simulink model "generico_f"  (R2015a)
settings: Solver=ode23tb  StartTime=0.0  StopTime=0.129  FixedStep=Ts  MaxStep=1e-5  RelTol=1e-4
values from neighbouring files (symbols this model uses):
  Tsc = 1/(fsw)    (= 0.0001)    [leer_ensayo_E3_f.m]    (also in leer_ensayo_E4_f.m; leer_ensayo_E5_f.m)
libraries: simulink x6
Description:
  | Three-Phase Asynchronous Drive with Sensor Control
  | 
  | This example shows how to control and analyze the operation of an
  | Asynchronous Machine (ASM) using sensored rotor field-oriented control.
  | The model shows the main electrical circuit, with three additional subsystems
  | containing the controls, measurements, and scopes.  The Controls subsystem
  | contains two controllers: one for the Grid-Side Converter (AC/DC) and one for
  | the Machine-Side Converter (DC/AC).  The Scopes subsystem contains two time
  | scopes: one for the Grid-Side Converter and one for the ASM. When the model
  | is executed, a Spectrum Analyzer opens and displays frequency data for the
  | A-Phase Supply Current.
  | 
  | 
  | 
  | Copyright 2008-2016 The MathWorks, Inc.
settings Model: Creator=MathWorks  LastModifiedBy=54265
settings SolverCC: PositivePriorityOrder=on  InsertRTBMode=Always
settings DataIOCC: FinalStateName=estado_sim  InitialState=estado_sim_ini  LimitDataPoints=off  SaveFinalState=on  SaveFormat=StructureWithTime  SaveOutput=off  SaveTime=off
settings OptimizationCC: ExpressionDepthLimit=2147483647  EfficientMapNaN2IntZero=off
settings DebuggingCC: UnderspecifiedInitializationDetection=Classic  MergeDetectMultiDrivingBlocksExec=none  SolverPrmCheckMsg=warning  MultiTaskRateTransMsg=warning  StateNameClashWarn=warning
settings HardwareCC: TargetLongLongMode=on  TargetIntDivRoundTo=Zero  TargetEndianess=LittleEndian  TargetHWDeviceType=MATLAB Host  ProdEqTarget=off
settings CodeAppCC: MaxIdLength=128
settings GRTTargetCC: CombineOutputUpdateFcns=off  GRTInterface=on

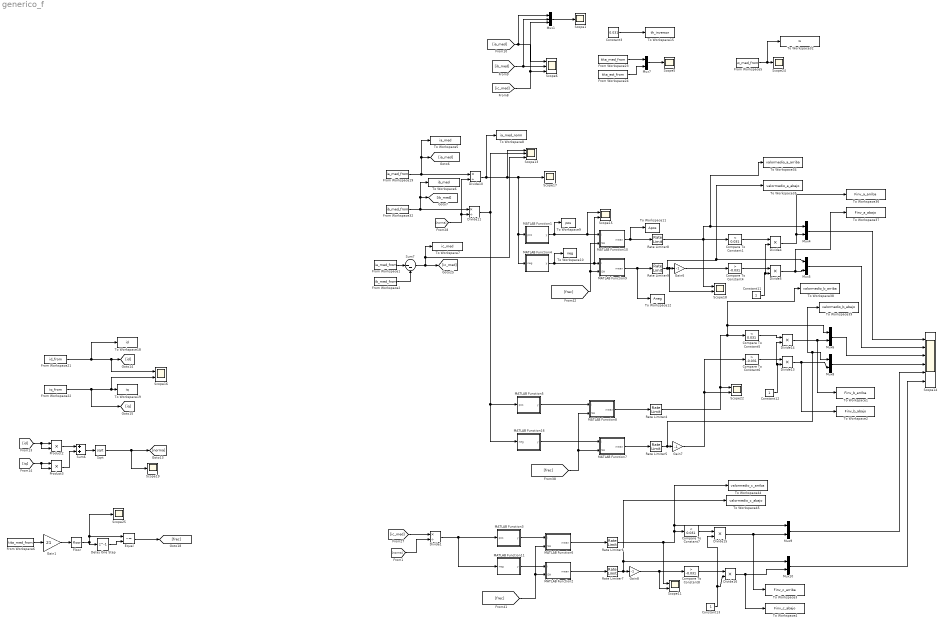
== system generico_f ==
  Compare To Constant1 : simulink/Logic and Bit Operations/Compare To Constant  relop=<  const=0.031  OutDataTypeStr=boolean
  Compare To Constant4 : simulink/Logic and Bit Operations/Compare To Constant  relop=>  const=-0.031  OutDataTypeStr=boolean
  Compare To Constant5 : simulink/Logic and Bit Operations/Compare To Constant  relop=<  const=0.031  OutDataTypeStr=boolean
  Compare To Constant6 : simulink/Logic and Bit Operations/Compare To Constant  relop=>  const=-0.031  OutDataTypeStr=boolean
  Compare To Constant7 : simulink/Logic and Bit Operations/Compare To Constant  relop=<  const=0.031  OutDataTypeStr=boolean
  Compare To Constant8 : simulink/Logic and Bit Operations/Compare To Constant  relop=>  const=-0.031  OutDataTypeStr=boolean
  Constant11 : Constant
  Constant12 : Constant
  Constant13 : Constant
  Constant3 : Constant  Value=0.031
  Delay One Step : Delay  DelayLength=1
  Divide1 : Product  Inputs=*/
  Divide10 : Product  Inputs=*/
  Divide11 : Product  Inputs=*/
  Divide{4..5,13..16} (6 alike) : Product  Inputs=**
  Equal : RelationalOperator  Operator=~=  OutDataTypeStr=boolean
  Floor : Rounding
  From Workspace1 : FromWorkspace  VariableName=ia_med_from  SampleTime=Tsc  OutputAfterFinalValue=Setting to zero
  From Workspace19 : FromWorkspace  VariableName=ia_med_from  SampleTime=Tsc  OutputAfterFinalValue=Setting to zero
  From Workspace2 : FromWorkspace  VariableName=ib_med_from  SampleTime=Tsc  OutputAfterFinalValue=Setting to zero
  From Workspace21 : FromWorkspace  VariableName=id_from  SampleTime=Tsc  OutputAfterFinalValue=Setting to zero
  From Workspace22 : FromWorkspace  VariableName=iq_from  SampleTime=Tsc  OutputAfterFinalValue=Setting to zero
  From Workspace23 : FromWorkspace  VariableName=tita_med_from  SampleTime=Tsc  OutputAfterFinalValue=Setting to zero
  From Workspace24 : FromWorkspace  VariableName=tita_est_from  SampleTime=Tsc  OutputAfterFinalValue=Setting to zero
  From Workspace32 : FromWorkspace  VariableName=ib_med_from  SampleTime=Tsc  OutputAfterFinalValue=Setting to zero
  From Workspace5 : FromWorkspace  VariableName=w_med_from  SampleTime=Tsc  OutputAfterFinalValue=Setting to zero
  From Workspace6 : FromWorkspace  VariableName=tita_med_from  SampleTime=Tsc  OutputAfterFinalValue=Setting to zero
  Gain1 : Gain  Gain=21
  Gain6 : Gain  Gain=-1
  Gain7 : Gain  Gain=-1
  Gain8 : Gain  Gain=-1
  MATLAB Function1 : MATLAB Function  TreatAsAtomicUnit=on
  MATLAB Function10 : MATLAB Function  TreatAsAtomicUnit=on
  MATLAB Function11 : MATLAB Function  TreatAsAtomicUnit=on
  MATLAB Function16 : MATLAB Function  TreatAsAtomicUnit=on
  MATLAB Function2 : MATLAB Function  TreatAsAtomicUnit=on
  MATLAB Function3 : MATLAB Function  TreatAsAtomicUnit=on
  MATLAB Function4 : MATLAB Function  TreatAsAtomicUnit=on
  MATLAB Function5 : MATLAB Function  TreatAsAtomicUnit=on
  MATLAB Function6 : MATLAB Function  TreatAsAtomicUnit=on
  MATLAB Function7 : MATLAB Function  TreatAsAtomicUnit=on
  MATLAB Function8 : MATLAB Function  TreatAsAtomicUnit=on
  MATLAB Function9 : MATLAB Function  TreatAsAtomicUnit=on
  Mux1 : Mux  Inputs=3
  Mux{4..10} (7 alike) : Mux  Inputs=2
  Product2 : Product
  Product3 : Product
  Rate Limiter{4..9} (6 alike) : RateLimiter  RisingSlewLimit=100000  FallingSlewLimit=-40
  Scope{1,5,17,19,24..25} (6 alike) : Scope
      Scope1 settings: TimeRange=1.2  YMin=0.6965  YMax=0.70025
      Scope17 settings: TimeRange=1.2  YMin=-1066.28  YMax=178.833  SaveName=ScopeData22
      Scope19 settings: TimeRange=1.2  YMin=-1066.28418  YMax=178.83301  SaveName=ScopeData21  Decimation=10
      Scope24 settings: TimeRange=0.129  YMin=0.45  YMax=0.55  SaveName=ScopeData28
      Scope25 settings: TimeRange=1.2  YMin=70.17554  YMax=98.54179  SaveName=ScopeData29  Decimation=10
      Scope5 settings: TimeRange=1.2  YMin=0.6965  YMax=0.70025  SaveName=ScopeData4  Decimation=10
  Scope{11,15..16,18,22} (5 alike) : Scope  NumInputPorts=2
      Scope11 settings: TimeRange=1.2  YMin=-1066.28~-5  YMax=178.833~5  SaveName=ScopeData11  Decimation=10
      Scope15 settings: TimeRange=1.2  YMin=-1066.28~-5  YMax=178.833~5  SaveName=ScopeData19
      Scope16 settings: TimeRange=1.2  YMin=-0.5~-5  YMax=1.5~5  SaveName=ScopeData18  Decimation=10
      Scope18 settings: TimeRange=1.2  YMin=-1066.28~-5  YMax=178.833~5  SaveName=ScopeData20  Decimation=10
      Scope22 settings: TimeRange=1.2  YMin=-1066.28~-5  YMax=178.833~5  SaveName=ScopeData6  Decimation=10
  Scope13 : Scope  NumInputPorts=3
      settings: TimeRange=1.2  YMin=-1066.28~-5~-5  YMax=178.833~5~5  SaveName=ScopeData14
  Scope14 : Scope  NumInputPorts=6
      settings: TimeRange=0.3075862068965519  YMin=0~0~0~0~0~0  YMax=0.952703~1~1~1~1~1  SaveName=ScopeData12  Decimation=2
  Scope6 : Scope  NumInputPorts=3
      settings: TimeRange=1.2  YMin=-0.5~-5~-5  YMax=1.5~5~5  SaveName=ScopeData5
  Sqrt : Sqrt  SaturateOnIntegerOverflow=on
  Sum6 : Sum
  Sum7 : Sum  Inputs=|--
  To Workspace1 : ToWorkspace  VariableName=Finv_b_arriba  SaveFormat=Timeseries  SampleTime=-1
  To Workspace10 : ToWorkspace  VariableName=neg  SaveFormat=Timeseries  SampleTime=Tsc
  To Workspace11 : ToWorkspace  VariableName=Apos  SaveFormat=Timeseries  SampleTime=Tsc
  To Workspace12 : ToWorkspace  VariableName=Aneg  SaveFormat=Timeseries  SampleTime=Tsc
  To Workspace15 : ToWorkspace  VariableName=th_inversor  SaveFormat=Timeseries  SampleTime=-1
  To Workspace18 : ToWorkspace  VariableName=id  SaveFormat=Timeseries  SampleTime=-1
  To Workspace19 : ToWorkspace  VariableName=iq  SaveFormat=Timeseries  SampleTime=-1
  To Workspace2 : ToWorkspace  VariableName=Finv_b_abajo  SaveFormat=Timeseries  SampleTime=-1
  To Workspace3 : ToWorkspace  VariableName=Finv_c_arriba  SaveFormat=Timeseries  SampleTime=-1
  To Workspace32 : ToWorkspace  VariableName=w  SaveFormat=Timeseries  SampleTime=Tsc
  To Workspace34 : ToWorkspace  VariableName=valormedio_a_arriba  SaveFormat=Timeseries  SampleTime=-1
  To Workspace35 : ToWorkspace  VariableName=valormedio_a_abajo  SaveFormat=Timeseries  SampleTime=-1
  To Workspace36 : ToWorkspace  VariableName=Finv_a_arriba  SaveFormat=Timeseries  SampleTime=-1
  To Workspace37 : ToWorkspace  VariableName=Finv_a_abajo  SaveFormat=Timeseries  SampleTime=-1
  To Workspace38 : ToWorkspace  VariableName=valormedio_b_arriba  SaveFormat=Timeseries  SampleTime=-1
  To Workspace39 : ToWorkspace  VariableName=valormedio_b_abajo  SaveFormat=Timeseries  SampleTime=-1
  To Workspace4 : ToWorkspace  VariableName=Finv_c_abajo  SaveFormat=Timeseries  SampleTime=-1
  To Workspace44 : ToWorkspace  VariableName=valormedio_c_arriba  SaveFormat=Timeseries  SampleTime=-1
  To Workspace45 : ToWorkspace  VariableName=valormedio_c_abajo  SaveFormat=Timeseries  SampleTime=-1
  To Workspace5 : ToWorkspace  VariableName=ia_med  SaveFormat=Timeseries  SampleTime=Tsc
  To Workspace6 : ToWorkspace  VariableName=ib_med  SaveFormat=Timeseries  SampleTime=Tsc
  To Workspace7 : ToWorkspace  VariableName=ic_med  SaveFormat=Timeseries  SampleTime=Tsc
  To Workspace8 : ToWorkspace  VariableName=ia_med_norm  SaveFormat=Timeseries  SampleTime=Tsc
  To Workspace9 : ToWorkspace  VariableName=pos  SaveFormat=Timeseries  SampleTime=Tsc
  wires:
  [id] -> Product2/2, Product2/1
  [iq] -> Product3/2, Product3/1
  Product2/1 -> Sum6/1
  Product3/1 -> Sum6/2
  Sum6/1 -> Sqrt/1
  Sqrt/1 -> Scope19/1, [norma]
  From Workspace21/1 -> Scope16/1, [id], To Workspace18/1
  From Workspace22/1 -> [iq], Scope16/2, To Workspace19/1
  From Workspace24/1 -> Mux7/2
  Mux7/1 -> Scope5/1
  From Workspace23/1 -> Mux7/1
  [norma] -> Divide10/2, Divide11/2
  From Workspace19/1 -> To Workspace5/1, [ia_med], Divide10/1
  MATLAB Function7/1(mean) -> Rate Limiter5/1
  MATLAB Function8/1(mean) -> Rate Limiter4/1
  Rate Limiter9/1 -> Mux5/1, To Workspace35/1, Scope18/2, Gain6/1
  Rate Limiter8/1 -> Mux4/1, To Workspace34/1, Compare To Constant1/1, Scope18/1
  Divide4/1 -> To Workspace36/1, Mux4/2
  Divide5/1 -> To Workspace37/1, Mux5/2
  Gain6/1 -> Compare To Constant4/1
  Rate Limiter4/1 -> Mux6/1, To Workspace38/1, Compare To Constant5/1, Scope22/1
  Gain7/1 -> Compare To Constant6/1, Scope22/2
  Rate Limiter5/1 -> Mux8/1, To Workspace39/1, Gain7/1
  MATLAB Function2/1(mean) -> Rate Limiter7/1
  MATLAB Function6/1(mean) -> Rate Limiter6/1
  Rate Limiter6/1 -> To Workspace44/1, Mux9/1, Compare To Constant7/1, Scope11/1
  Gain8/1 -> Compare To Constant8/1, Scope11/2
  Rate Limiter7/1 -> Mux10/1, To Workspace45/1, Gain8/1
  Compare To Constant1/1 -> Divide4/1
  Constant11/1 -> Divide4/2, Divide5/2
  Compare To Constant4/1 -> Divide5/1
  Compare To Constant6/1 -> Divide13/1
  Constant12/1 -> Divide14/2, Divide13/2
  Compare To Constant5/1 -> Divide14/1
  Compare To Constant7/1 -> Divide15/1
  Constant13/1 -> Divide16/2, Divide15/2
  Compare To Constant8/1 -> Divide16/1
  Mux5/1 -> Scope14/2
  Divide14/1 -> To Workspace1/1, Mux6/2
  Divide13/1 -> To Workspace2/1, Mux8/2
  Mux6/1 -> Scope14/3
  Mux8/1 -> Scope14/4
  Divide16/1 -> To Workspace4/1, Mux10/2
  Divide15/1 -> To Workspace3/1, Mux9/2
  Mux9/1 -> Scope14/5
  Mux10/1 -> Scope14/6
  [ib_med] -> Mux1/2, Scope6/2
  [ia_med] -> Mux1/1, Scope6/1
  [ic_med] -> Mux1/3, Scope6/3
  Mux4/1 -> Scope14/1
  Divide11/1 -> MATLAB Function16/1(neg), MATLAB Function5/1(pos), Scope13/2
  Divide10/1 -> To Workspace8/1, Scope17/1, MATLAB Function4/1(neg), MATLAB Function1/1(pos), Scope13/1
  Sum7/1 -> To Workspace7/1, Scope13/3, [ic_med]
  Divide1/1 -> MATLAB Function11/1(neg), MATLAB Function3/1(pos)
  From Workspace6/1 -> Gain1/1
  Gain1/1 -> Floor/1
  Delay One Step/1 -> Equal/2
  Floor/1 -> Scope25/1, Equal/1, Delay One Step/1
  Equal/1 -> [frec]
  [frec] -> MATLAB Function6/2(SH), MATLAB Function2/2(SH)
  [frec] -> MATLAB Function8/2(SH), MATLAB Function7/2(SH)
  MATLAB Function9/1(mean) -> To Workspace12/1, Rate Limiter9/1
  MATLAB Function10/1(mean) -> To Workspace11/1, Rate Limiter8/1
  [frec] -> MATLAB Function10/2(SH), MATLAB Function9/2(SH)
  From Workspace5/1 -> To Workspace32/1, Scope24/1
  From Workspace32/1 -> To Workspace6/1, [ib_med], Divide11/1
  Mux1/1 -> Scope1/1
  From Workspace1/1 -> Sum7/1
  From Workspace2/1 -> Sum7/2
  [norma] -> Divide1/2
  [ic_med] -> Divide1/1
  Constant3/1 -> To Workspace15/1
  MATLAB Function4/1(y) -> Scope15/2, MATLAB Function9/1(i), To Workspace10/1
  MATLAB Function1/1(y) -> To Workspace9/1, Scope15/1, MATLAB Function10/1(i)
  MATLAB Function16/1(y) -> MATLAB Function7/1(i)
  MATLAB Function5/1(y) -> MATLAB Function8/1(i)
  MATLAB Function11/1(y) -> MATLAB Function2/1(i)
  MATLAB Function3/1(y) -> MATLAB Function6/1(i)

== matlab function generico_f/MATLAB Function1 ==
  data: pos input; y output
function y = fcn(pos)

if (pos>0);
pos = pos;

else
    
pos = 0;

end

y = pos;

== matlab function generico_f/MATLAB Function2 ==
  data: i input; mean output; SH input
function mean   = fcn(i, SH)

N=21;

persistent ia_buff;
persistent n;
persistent mean_s;
persistent SH_prev;
persistent test;

%% Inicializaciones    
if isempty(ia_buff)
    ia_buff = zeros(N,1);
end

if isempty(n)
    n = 1;
end

if isempty(mean_s)
    mean_s = 0.0;
end

if isempty(SH_prev)
    SH_prev = 0;
end

if isempty(test)
    test = 0;
end

%% Mean 

if (SH == 1) %&& (SH_prev == 0) 
    %ia_buff(n) = i;
    test = i;
    if n >= N
        mean_s = mean_s + (i - ia_buff(1))/N;
        n = 1;
    else
        mean_s = mean_s + (i - ia_buff(n+1))/N;
        n = n+1;
    end 
    ia_buff(n) = i;
end

SH_prev = double(SH) ;

%% Salida
mean = mean_s;

== matlab function generico_f/MATLAB Function6 ==
  data: i input; mean output; SH input
function mean   = fcn(i, SH)

N=21;

persistent ia_buff;
persistent n;
persistent mean_s;
persistent SH_prev;
persistent test;

%% Inicializaciones    
if isempty(ia_buff)
    ia_buff = zeros(N,1);
end

if isempty(n)
    n = 1;
end

if isempty(mean_s)
    mean_s = 0.0;
end

if isempty(SH_prev)
    SH_prev = 0;
end

if isempty(test)
    test = 0;
end

%% Mean 

if (SH == 1) %&& (SH_prev == 0) 
    %ia_buff(n) = i;
    test = i;
    if n >= N
        mean_s = mean_s + (i - ia_buff(1))/N;
        n = 1;
    else
        mean_s = mean_s + (i - ia_buff(n+1))/N;
        n = n+1;
    end 
    ia_buff(n) = i;
end

SH_prev = double(SH) ;

%% Salida
mean = mean_s;

== matlab function generico_f/MATLAB Function7 ==
  data: i input; mean output; SH input
function mean   = fcn(i, SH)

N=21;

persistent ia_buff;
persistent n;
persistent mean_s;
persistent SH_prev;
persistent test;

%% Inicializaciones    
if isempty(ia_buff)
    ia_buff = zeros(N,1);
end

if isempty(n)
    n = 1;
end

if isempty(mean_s)
    mean_s = 0.0;
end

if isempty(SH_prev)
    SH_prev = 0;
end

if isempty(test)
    test = 0;
end

%% Mean 

if (SH == 1) %&& (SH_prev == 0) 
    %ia_buff(n) = i;
    test = i;
    if n >= N
        mean_s = mean_s + (i - ia_buff(1))/N;
        n = 1;
    else
        mean_s = mean_s + (i - ia_buff(n+1))/N;
        n = n+1;
    end 
    ia_buff(n) = i;
end

SH_prev = double(SH) ;

%% Salida
mean = mean_s;

== matlab function generico_f/MATLAB Function4 ==
  data: neg input; y output
function y = fcn(neg)

if (neg<0);
neg = -neg;

else
    
neg = 0;

end

y = neg;

== matlab function generico_f/MATLAB Function16 ==
  data: neg input; y output
function y = fcn(neg)

if (neg<0);
neg = -neg;

else
    
neg = 0;

end

y = neg;

== matlab function generico_f/MATLAB Function5 ==
  data: pos input; y output
function y = fcn(pos)

if (pos>0);
pos = pos;

else
    
pos = 0;

end

y = pos;

== matlab function generico_f/MATLAB Function3 ==
  data: pos input; y output
function y = fcn(pos)

if (pos>0);
pos = pos;

else
    
pos = 0;

end

y = pos;

== matlab function generico_f/MATLAB Function11 ==
  data: neg input; y output
function y = fcn(neg)

if (neg<0);
neg = -neg;

else
    
neg = 0;

end

y = neg;

== matlab function generico_f/MATLAB Function8 ==
  data: i input; mean output; SH input
function mean   = fcn(i, SH)

N=21;

persistent ia_buff;
persistent n;
persistent mean_s;
persistent SH_prev;
persistent test;

%% Inicializaciones    
if isempty(ia_buff)
    ia_buff = zeros(N,1);
end

if isempty(n)
    n = 1;
end

if isempty(mean_s)
    mean_s = 0.0;
end

if isempty(SH_prev)
    SH_prev = 0;
end

if isempty(test)
    test = 0;
end

%% Mean 

if (SH == 1) %&& (SH_prev == 0) 
    %ia_buff(n) = i;
    test = i;
    if n >= N
        mean_s = mean_s + (i - ia_buff(1))/N;
        n = 1;
    else
        mean_s = mean_s + (i - ia_buff(n+1))/N;
        n = n+1;
    end 
    ia_buff(n) = i;
end

SH_prev = double(SH) ;

%% Salida
mean = mean_s;

== matlab function generico_f/MATLAB Function10 ==
  data: i input; mean output; SH input
function mean   = fcn(i, SH)

N=21;

persistent ia_buff;
persistent n;
persistent mean_s;
persistent SH_prev;
persistent test;

%% Inicializaciones    
if isempty(ia_buff)
    ia_buff = zeros(N,1);
end

if isempty(n)
    n = 1;
end

if isempty(mean_s)
    mean_s = 0.0;
end

if isempty(SH_prev)
    SH_prev = 0;
end

if isempty(test)
    test = 0;
end

%% Mean 

if (SH == 1) %&& (SH_prev == 0) 
    %ia_buff(n) = i;
    test = i;
    if n >= N
        mean_s = mean_s + (i - ia_buff(1))/N;
        n = 1;
    else
        mean_s = mean_s + (i - ia_buff(n+1))/N;
        n = n+1;
    end 
    ia_buff(n) = i;
end

SH_prev = double(SH) ;

%% Salida
mean = mean_s;

== matlab function generico_f/MATLAB Function9 ==
  data: i input; mean output; SH input
function mean   = fcn(i, SH)

N=21;

persistent ia_buff;
persistent n;
persistent mean_s;
persistent SH_prev;
persistent test;

%% Inicializaciones    
if isempty(ia_buff)
    ia_buff = zeros(N,1);
end

if isempty(n)
    n = 1;
end

if isempty(mean_s)
    mean_s = 0.0;
end

if isempty(SH_prev)
    SH_prev = 0;
end

if isempty(test)
    test = 0;
end

%% Mean 

if (SH == 1) %&& (SH_prev == 0) 
    %ia_buff(n) = i;
    test = i;
    if n >= N
        mean_s = mean_s + (i - ia_buff(1))/N;
        n = 1;
    else
        mean_s = mean_s + (i - ia_buff(n+1))/N;
        n = n+1;
    end 
    ia_buff(n) = i;
end

SH_prev = double(SH) ;

%% Salida
mean = mean_s;
